simulink model "simulation"  (R2022b)
settings: Solver=VariableStepAuto  StartTime=0.0  StopTime=0.1  MaxStep=0.001  RelTol=1e-3
values from neighbouring files (symbols this model uses):
  d = 0.396    [parameters.m]
  Lmin = 1.29e-3    (= 0.00129)    [parameters.m]
  m = 8.5e-3    (= 0.0085)    [parameters.m]
  R = 2    [parameters.m]
  z0 = -10.51e-3    (= -0.01051)    [parameters.m]
  zs = 9.60e-3    (= 0.0096)    [parameters.m]
libraries: slpidlib x1
settings Model: Creator=Fabian Mink  LastModifiedBy=Fabian Mink

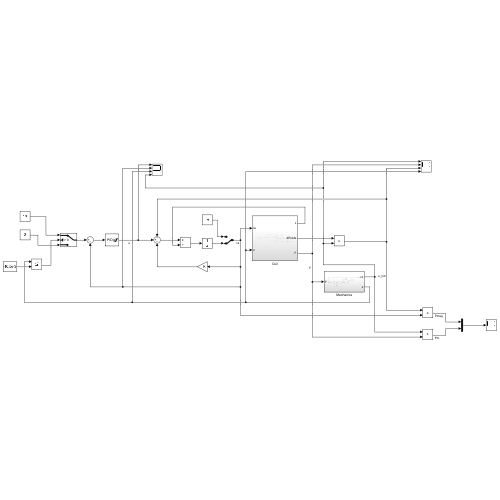
[thumbnail: Simulink's stored preview of the top-level diagram]
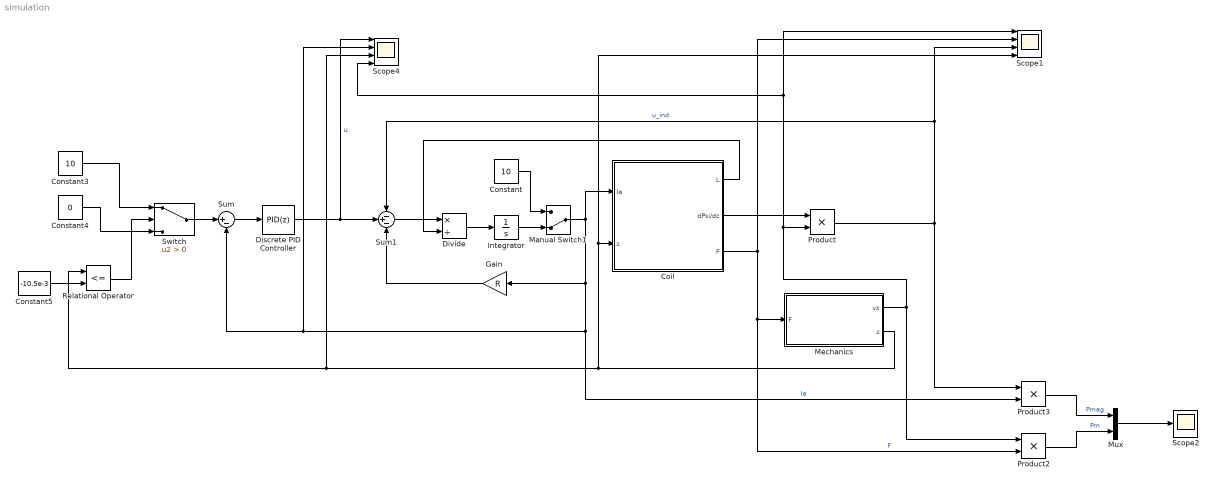
== system simulation ==
  Coil : Subsystem
  Constant : Constant  Value=10
  Constant3 : Constant  Value=10
  Constant4 : Constant  Value=0
  Constant5 : Constant  Value=-10.5e-3
  Discrete PID Controller : slpidlib/PID Controller  Controller=PID  Form=Parallel  TimeDomain=Discrete-time  UseExternalTs=off  SampleTime=62.5e-6  IntegratorMethod=Forward Euler  FilterMethod=Forward Euler  ControllerParametersSource=internal  P=5  I=5/0.001  UseKiTs=off  D=0  N=100  UseFilter=on  TunerSelectOption=Transfer Function Based (PID Tuner App)  InitialConditionSource=internal  InitialConditionForIntegrator=0  InitialConditionForFilter=0  DifferentiatorICPrevScaledInput=0  ExternalReset=none  TrackingMode=off  Kt=1  LimitOutput=on  SatLimitsSource=internal  UpperSaturationLimit=24  LowerSaturationLimit=-24  LinearizeAsGain=off  AntiWindupMode=clamping  Kb=1  LimitIntegrator=off  UpperIntegratorSaturationLimit=inf  LowerIntegratorSaturationLimit=-inf  POutMin=[]  POutMax=[]  IOutMin=[]  IOutMax=[]  DOutMin=[]  DOutMax=[]  NOutMin=[]  NOutMax=[]  SumOutMin=[]  SumOutMax=[]  SaturationOutMin=[]  SaturationOutMax=[]  PParamMin=[]  PParamMax=[]  IParamMin=[]  IParamMax=[]  DParamMin=[]  DParamMax=[]  NParamMin=[]  NParamMax=[]  KbParamMin=[]  KbParamMax=[]  KtParamMin=[]  KtParamMax=[]  KbOutMin=[]  KbOutMax=[]  KtOutMin=[]  KtOutMax=[]  IntegratorOutMin=[]  IntegratorOutMax=[]  FilterOutMin=[]  FilterOutMax=[]  SumI1OutMin=[]  SumI1OutMax=[]  SumI2OutMin=[]  SumI2OutMax=[]  SumI3OutMin=[]  SumI3OutMax=[]  SumI4OutMin=[]  SumI4OutMax=[]  SumDOutMin=[]  SumDOutMax=[]  DifferentiatorOutMin=[]  DifferentiatorOutMax=[]  FilterDiffOutCoefMin=[]  FilterDiffOutCoefMax=[]  ReciprocalOutMin=[]  ReciprocalOutMax=[]  SumDenOutMin=[]  SumDenOutMax=[]  SumNumOutMin=[]  SumNumOutMax=[]  DivideOutMin=[]  DivideOutMax=[]  UdiffTsProdOutMin=[]  UdiffTsProdOutMax=[]  NTsProdOutMin=[]  NTsProdOutMax=[]  UintegralTsProdOutMin=[]  UintegralTsProdOutMax=[]  UngainTsProdOutMin=[]  UngainTsProdOutMax=[]  ClampingZeroOutDataTypeStr=Inherit: Inherit via back propagation  ClampingZeroOutMin=[]  ClampingZeroOutMax=[]  FilterDenConstantOutDataTypeStr=Inherit: Inherit via back propagation  FilterDenConstantOutMin=[]  FilterDenConstantOutMax=[]  PCopyOutDataTypeStr=Inherit: Inherit via back propagation  PCopyOutMin=[]  PCopyOutMax=[]  NCopyOutDataTypeStr=Inherit: Inherit via back propagation  NCopyOutMin=[]  NCopyOutMax=[]  IntegratorContinuousStateAttributes=''  IntegratorStateMustResolveToSignalObject=off  IntegratorRTWStateStorageClass=Auto  FilterContinuousStateAttributes=''  FilterStateMustResolveToSignalObject=off  FilterRTWStateStorageClass=Auto  ParallelPVariant=InternalParameters  IdealPVariant=Disabled  IVariant=InternalParameters  DVariant=InternalParameters  IntegratorVariant=Discrete  SatVariant=Enabled  AWVariant=DiscClampingParallel  PCopyVariant=Disabled  TRVariant=Disabled  FdbkBlocksVariant=Forward  IdealPFdbkVariant=Disabled  SatFdbkVariant=Disabled  DerivativeFilterVariant=ForwardEulerFilter  NVariant=InternalParameters  NCopyVariant=Disabled  FilterICVariant=InternalICsFilter  IntegratorICVariant=InternalICs  ExternalResetVariant=Disabled  TRSumVariant=Passthrough  SumFdbkVariant=Disabled  SumVariant=Sum_PID  TsampFilterVariant=InternalTs  TsampNgainVariant=Passthrough  TsampIntegralVariant=Passthrough  ExternalSaturationOutDataTypeStr=Inherit: Same as second input
      settings: LibrarySourceBlock=simulink/Discrete/Discrete PID Controller
  Divide : Product  Inputs=*/
  Gain : Gain  Gain=R
  Integrator : Integrator
  Manual Switch1 : ManualSwitch  CurrentSetting=0
  Mechanics : Subsystem
  Mux : Mux  Inputs=2
  Product : Product
  Product2 : Product
  Product3 : Product
  Relational Operator : RelationalOperator  Operator=<=  OutDataTypeStr=boolean  RndMeth=Simplest  InputSameDT=off
  Scope1 : Scope  NumInputPorts=4
  Scope2 : Scope
  Scope4 : Scope  NumInputPorts=4
  Sum : Sum  Inputs=|+-
  Sum1 : Sum  Inputs=-+-
  Switch : Switch  Criteria=u2 > Threshold  SaturateOnIntegerOverflow=off  InputSameDT=off
  wires:
  Manual Switch1/1 -> Scope4/2, Sum/2, Product3/2, Gain/1, Coil/1(Ia)  "Ia"
  Coil/3(F) -> Product2/2, Mechanics/1(F), Scope1/2  "F"
  Coil/2(dPsi/dz) -> Product/1
  Product/1 -> Product3/1, Sum1/1, Scope1/3  "u_ind"
  Mux/1 -> Scope2/1
  Product3/1 -> Mux/1  "Pmag"
  Product2/1 -> Mux/2  "Pm"
  Constant/1 -> Manual Switch1/1
  Constant3/1 -> Switch/1
  Relational Operator/1 -> Switch/2
  Constant4/1 -> Switch/3
  Sum/1 -> Discrete PID Controller/1
  Switch/1 -> Sum/1
  Mechanics/2(z) -> Relational Operator/1, Scope4/3, Coil/2(z), Scope1/4
  Mechanics/1(vz) -> Product2/1, Product/2, Scope4/4, Scope1/1
  Integrator/1 -> Manual Switch1/2
  Divide/1 -> Integrator/1
  Coil/1(L) -> Divide/2
  Sum1/1 -> Divide/1
  Gain/1 -> Sum1/3
  Discrete PID Controller/1 -> Scope4/1, Sum1/2  "u"
  Constant5/1 -> Relational Operator/2

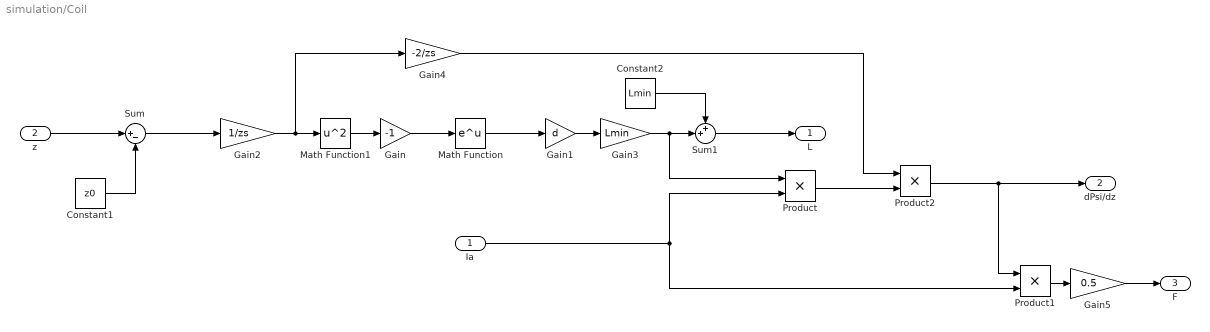
== system simulation/Coil ==
  Ia : Inport
  z : Inport  Port=2
  Constant1 : Constant  Value=z0
  Constant2 : Constant  Value=Lmin
  Gain : Gain  Gain=-1
  Gain1 : Gain  Gain=d
  Gain2 : Gain  Gain=1/zs
  Gain3 : Gain  Gain=Lmin
  Gain4 : Gain  Gain=-2/zs
  Gain5 : Gain  Gain=0.5
  Math Function : Math
  Math Function1 : Math  Operator=square
  Product : Product
  Product1 : Product
  Product2 : Product
  Sum : Sum  Inputs=|+-
  Sum1 : Sum  Inputs=++|
  L : Outport
  dPsi/dz : Outport  Port=2
  F : Outport  Port=3
  wires:
  Sum/1 -> Gain2/1
  Math Function1/1 -> Gain/1
  Gain2/1 -> Gain4/1, Math Function1/1
  Math Function/1 -> Gain1/1
  Gain/1 -> Math Function/1
  Constant1/1 -> Sum/2
  z/1 -> Sum/1
  Ia/1 -> Product1/2, Product/2
  Product2/1 -> Product1/1, dPsi/dz/1
  Product1/1 -> Gain5/1
  Gain5/1 -> F/1
  Constant2/1 -> Sum1/1
  Gain1/1 -> Gain3/1
  Gain3/1 -> Product/1, Sum1/2
  Sum1/1 -> L/1
  Product/1 -> Product2/2
  Gain4/1 -> Product2/1

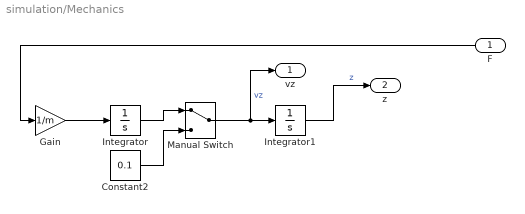
== system simulation/Mechanics ==
  F : Inport
  Constant2 : Constant  Value=0.1
  Gain : Gain  Gain=1/m
  Integrator : Integrator
  Integrator1 : Integrator  InitialCondition=-30e-3
  Manual Switch : ManualSwitch
  vz : Outport
  z : Outport  Port=2
  wires:
  Integrator/1 -> Manual Switch/1
  Constant2/1 -> Manual Switch/2
  F/1 -> Gain/1
  Gain/1 -> Integrator/1
  Manual Switch/1 -> vz/1, Integrator1/1  "vz"
  Integrator1/1 -> z/1  "z"
